simulink model "full_car_model"  (Simulink 7.0)
settings: Solver=ode45  StartTime=0.0  StopTime=120  RelTol=1e-3
values from neighbouring files (symbols this model uses):
  M = 0.02897    [CalculateTireWeight.m]    (also in SimFunc.m = [M11 M12; matrix_main.m)
undefined symbols (not defined in the file or in its folder): a, b, c, c01, c02, c03, c04, c1, c2, c3, c4, d, Ix, Iy, k01, k02, k03, k04, k1, k2, k3, k4, m1, m2, m3, m4, sigbuilder_block
(part 2 of 2)

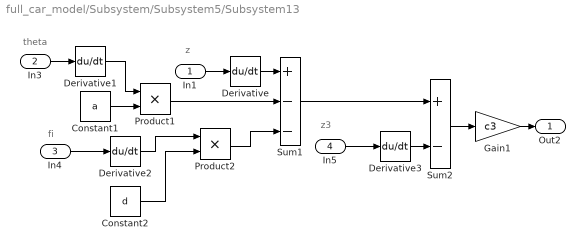
== system full_car_model/Subsystem/Subsystem5/Subsystem13 ==
  note: z3
  note: fi
  note: theta
  note: z
  In1 : Inport  OutDataType=sfix(16)  OutScaling=2^0
  In3 : Inport  Port=2  OutDataType=sfix(16)  OutScaling=2^0
  In4 : Inport  Port=3  OutDataType=sfix(16)  OutScaling=2^0
  In5 : Inport  Port=4  OutDataType=sfix(16)  OutScaling=2^0
  Constant1 : Constant  Value=a  OutDataType=sfix(16)  OutScaling=2^0
  Constant2 : Constant  Value=d  OutDataType=sfix(16)  OutScaling=2^0
  Derivative{,1..3} (4 alike) : Derivative
  Gain1 : Gain  Gain=c3  ParameterDataType=sfix(16)  ParameterScaling=2^0  OutDataType=sfix(16)  OutScaling=2^0
  Product1 : Product  OutDataType=sfix(16)  OutScaling=2^0  RndMeth=Zero
  Product2 : Product  OutDataType=sfix(16)  OutScaling=2^0  RndMeth=Zero
  Sum1 : Sum  Inputs=+--  OutDataType=sfix(16)  OutScaling=2^0
  Sum2 : Sum  Inputs=+-  OutDataType=sfix(16)  OutScaling=2^0
  Out2 : Outport  OutDataType=sfix(16)  OutScaling=2^0
  wires:
  Derivative2/1 -> Product2/1
  Derivative1/1 -> Product1/1
  Derivative/1 -> Sum1/1
  Gain1/1 -> Out2/1
  Product2/1 -> Sum1/3
  In5/1 -> Derivative3/1
  Constant2/1 -> Product2/2
  Product1/1 -> Sum1/2
  Constant1/1 -> Product1/2
  In4/1 -> Derivative2/1
  In3/1 -> Derivative1/1
  In1/1 -> Derivative/1
  Sum1/1 -> Sum2/1
  Derivative3/1 -> Sum2/2
  Sum2/1 -> Gain1/1

== system full_car_model/Subsystem/Subsystem6/Subsystem14 ==
  note: z4
  note: fi
  note: theta
  note: z
  In1 : Inport  OutDataType=sfix(16)  OutScaling=2^0
  In3 : Inport  Port=2  OutDataType=sfix(16)  OutScaling=2^0
  In4 : Inport  Port=3  OutDataType=sfix(16)  OutScaling=2^0
  In5 : Inport  Port=4  OutDataType=sfix(16)  OutScaling=2^0
  Constant1 : Constant  Value=b  OutDataType=sfix(16)  OutScaling=2^0
  Constant2 : Constant  Value=d  OutDataType=sfix(16)  OutScaling=2^0
  Gain1 : Gain  Gain=k4  ParameterDataType=sfix(16)  ParameterScaling=2^0  OutDataType=sfix(16)  OutScaling=2^0
  Product1 : Product  OutDataType=sfix(16)  OutScaling=2^0  RndMeth=Zero
  Product2 : Product  OutDataType=sfix(16)  OutScaling=2^0  RndMeth=Zero
  Sum1 : Sum  Inputs=++-  OutDataType=sfix(16)  OutScaling=2^0
  Sum2 : Sum  Inputs=+-  OutDataType=sfix(16)  OutScaling=2^0
  Out2 : Outport  OutDataType=sfix(16)  OutScaling=2^0
  wires:
  Gain1/1 -> Out2/1
  Product2/1 -> Sum1/3
  Constant2/1 -> Product2/2
  Product1/1 -> Sum1/2
  Constant1/1 -> Product1/2
  In4/1 -> Product2/1
  In3/1 -> Product1/1
  In1/1 -> Sum1/1
  Sum1/1 -> Sum2/1
  In5/1 -> Sum2/2
  Sum2/1 -> Gain1/1

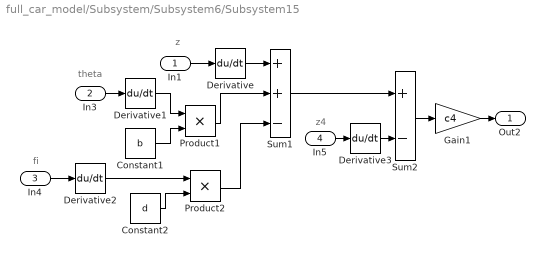
== system full_car_model/Subsystem/Subsystem6/Subsystem15 ==
  note: z
  note: theta
  note: fi
  note: z4
  In1 : Inport  OutDataType=sfix(16)  OutScaling=2^0
  In3 : Inport  Port=2  OutDataType=sfix(16)  OutScaling=2^0
  In4 : Inport  Port=3  OutDataType=sfix(16)  OutScaling=2^0
  In5 : Inport  Port=4  OutDataType=sfix(16)  OutScaling=2^0
  Constant1 : Constant  Value=b  OutDataType=sfix(16)  OutScaling=2^0
  Constant2 : Constant  Value=d  OutDataType=sfix(16)  OutScaling=2^0
  Derivative{,1..3} (4 alike) : Derivative
  Gain1 : Gain  Gain=c4  ParameterDataType=sfix(16)  ParameterScaling=2^0  OutDataType=sfix(16)  OutScaling=2^0
  Product1 : Product  OutDataType=sfix(16)  OutScaling=2^0  RndMeth=Zero
  Product2 : Product  OutDataType=sfix(16)  OutScaling=2^0  RndMeth=Zero
  Sum1 : Sum  Inputs=++-  OutDataType=sfix(16)  OutScaling=2^0
  Sum2 : Sum  Inputs=+-  OutDataType=sfix(16)  OutScaling=2^0
  Out2 : Outport  OutDataType=sfix(16)  OutScaling=2^0
  wires:
  Derivative2/1 -> Product2/1
  Derivative1/1 -> Product1/1
  Derivative/1 -> Sum1/1
  In1/1 -> Derivative/1
  In3/1 -> Derivative1/1
  In4/1 -> Derivative2/1
  Constant1/1 -> Product1/2
  Product1/1 -> Sum1/2
  Constant2/1 -> Product2/2
  In5/1 -> Derivative3/1
  Product2/1 -> Sum1/3
  Gain1/1 -> Out2/1
  Sum1/1 -> Sum2/1
  Derivative3/1 -> Sum2/2
  Sum2/1 -> Gain1/1

== system full_car_model/Subsystem1/Subsystem10/Subsystem20 ==
  note: z4
  note: fi
  note: theta
  note: z
  In1 : Inport  OutDataType=sfix(16)  OutScaling=2^0
  In3 : Inport  Port=2  OutDataType=sfix(16)  OutScaling=2^0
  In4 : Inport  Port=3  OutDataType=sfix(16)  OutScaling=2^0
  In5 : Inport  Port=4  OutDataType=sfix(16)  OutScaling=2^0
  Constant1 : Constant  Value=b  OutDataType=sfix(16)  OutScaling=2^0
  Constant2 : Constant  Value=d  OutDataType=sfix(16)  OutScaling=2^0
  Gain1 : Gain  Gain=k4  ParameterDataType=sfix(16)  ParameterScaling=2^0  OutDataType=sfix(16)  OutScaling=2^0
  Product1 : Product  OutDataType=sfix(16)  OutScaling=2^0  RndMeth=Zero
  Product2 : Product  OutDataType=sfix(16)  OutScaling=2^0  RndMeth=Zero
  Sum1 : Sum  Inputs=++-  OutDataType=sfix(16)  OutScaling=2^0
  Sum2 : Sum  Inputs=+-  OutDataType=sfix(16)  OutScaling=2^0
  Out2 : Outport  OutDataType=sfix(16)  OutScaling=2^0
  wires:
  Gain1/1 -> Out2/1
  Product2/1 -> Sum1/3
  Constant2/1 -> Product2/2
  Product1/1 -> Sum1/2
  Constant1/1 -> Product1/2
  In4/1 -> Product2/1
  In3/1 -> Product1/1
  In1/1 -> Sum1/1
  Sum1/1 -> Sum2/1
  In5/1 -> Sum2/2
  Sum2/1 -> Gain1/1

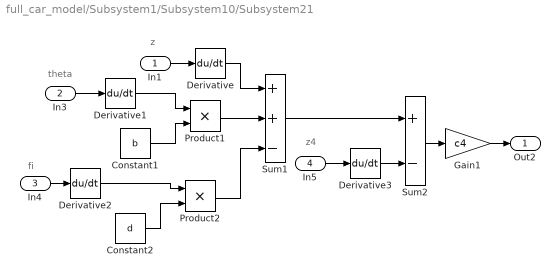
== system full_car_model/Subsystem1/Subsystem10/Subsystem21 ==
  note: z
  note: theta
  note: fi
  note: z4
  In1 : Inport  OutDataType=sfix(16)  OutScaling=2^0
  In3 : Inport  Port=2  OutDataType=sfix(16)  OutScaling=2^0
  In4 : Inport  Port=3  OutDataType=sfix(16)  OutScaling=2^0
  In5 : Inport  Port=4  OutDataType=sfix(16)  OutScaling=2^0
  Constant1 : Constant  Value=b  OutDataType=sfix(16)  OutScaling=2^0
  Constant2 : Constant  Value=d  OutDataType=sfix(16)  OutScaling=2^0
  Derivative{,1..3} (4 alike) : Derivative
  Gain1 : Gain  Gain=c4  ParameterDataType=sfix(16)  ParameterScaling=2^0  OutDataType=sfix(16)  OutScaling=2^0
  Product1 : Product  OutDataType=sfix(16)  OutScaling=2^0  RndMeth=Zero
  Product2 : Product  OutDataType=sfix(16)  OutScaling=2^0  RndMeth=Zero
  Sum1 : Sum  Inputs=++-  OutDataType=sfix(16)  OutScaling=2^0
  Sum2 : Sum  Inputs=+-  OutDataType=sfix(16)  OutScaling=2^0
  Out2 : Outport  OutDataType=sfix(16)  OutScaling=2^0
  wires:
  Derivative2/1 -> Product2/1
  Derivative1/1 -> Product1/1
  Derivative/1 -> Sum1/1
  In1/1 -> Derivative/1
  In3/1 -> Derivative1/1
  In4/1 -> Derivative2/1
  Constant1/1 -> Product1/2
  Product1/1 -> Sum1/2
  Constant2/1 -> Product2/2
  In5/1 -> Derivative3/1
  Product2/1 -> Sum1/3
  Gain1/1 -> Out2/1
  Sum1/1 -> Sum2/1
  Derivative3/1 -> Sum2/2
  Sum2/1 -> Gain1/1

== system full_car_model/Subsystem1/Subsystem7/Subsystem22 ==
  note: z1
  note: fi
  note: theta
  note: z
  In1 : Inport  OutDataType=sfix(16)  OutScaling=2^0
  In3 : Inport  Port=2  OutDataType=sfix(16)  OutScaling=2^0
  In4 : Inport  Port=3  OutDataType=sfix(16)  OutScaling=2^0
  In5 : Inport  Port=4  OutDataType=sfix(16)  OutScaling=2^0
  Constant1 : Constant  Value=a  OutDataType=sfix(16)  OutScaling=2^0
  Constant2 : Constant  Value=c  OutDataType=sfix(16)  OutScaling=2^0
  Gain1 : Gain  Gain=k1  ParameterDataType=sfix(16)  ParameterScaling=2^0  OutDataType=sfix(16)  OutScaling=2^0
  Product1 : Product  OutDataType=sfix(16)  OutScaling=2^0  RndMeth=Zero
  Product2 : Product  OutDataType=sfix(16)  OutScaling=2^0  RndMeth=Zero
  Sum1 : Sum  Inputs=+-+  OutDataType=sfix(16)  OutScaling=2^0
  Sum2 : Sum  Inputs=+-  OutDataType=sfix(16)  OutScaling=2^0
  Out2 : Outport  OutDataType=sfix(16)  OutScaling=2^0
  wires:
  Gain1/1 -> Out2/1
  Product2/1 -> Sum1/3
  Constant2/1 -> Product2/2
  Product1/1 -> Sum1/2
  Constant1/1 -> Product1/2
  In4/1 -> Product2/1
  In3/1 -> Product1/1
  In1/1 -> Sum1/1
  Sum1/1 -> Sum2/1
  In5/1 -> Sum2/2
  Sum2/1 -> Gain1/1

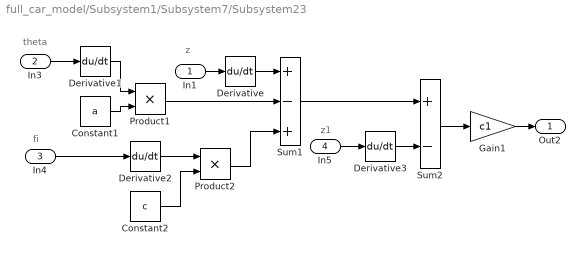
== system full_car_model/Subsystem1/Subsystem7/Subsystem23 ==
  note: z
  note: theta
  note: fi
  note: z1
  In1 : Inport  OutDataType=sfix(16)  OutScaling=2^0
  In3 : Inport  Port=2  OutDataType=sfix(16)  OutScaling=2^0
  In4 : Inport  Port=3  OutDataType=sfix(16)  OutScaling=2^0
  In5 : Inport  Port=4  OutDataType=sfix(16)  OutScaling=2^0
  Constant1 : Constant  Value=a  OutDataType=sfix(16)  OutScaling=2^0
  Constant2 : Constant  Value=c  OutDataType=sfix(16)  OutScaling=2^0
  Derivative{,1..3} (4 alike) : Derivative
  Gain1 : Gain  Gain=c1  ParameterDataType=sfix(16)  ParameterScaling=2^0  OutDataType=sfix(16)  OutScaling=2^0
  Product1 : Product  OutDataType=sfix(16)  OutScaling=2^0  RndMeth=Zero
  Product2 : Product  OutDataType=sfix(16)  OutScaling=2^0  RndMeth=Zero
  Sum1 : Sum  Inputs=+-+  OutDataType=sfix(16)  OutScaling=2^0
  Sum2 : Sum  Inputs=+-  OutDataType=sfix(16)  OutScaling=2^0
  Out2 : Outport  OutDataType=sfix(16)  OutScaling=2^0
  wires:
  Derivative2/1 -> Product2/1
  Derivative1/1 -> Product1/1
  Derivative/1 -> Sum1/1
  In1/1 -> Derivative/1
  In3/1 -> Derivative1/1
  In4/1 -> Derivative2/1
  Constant1/1 -> Product1/2
  Product1/1 -> Sum1/2
  Constant2/1 -> Product2/2
  In5/1 -> Derivative3/1
  Product2/1 -> Sum1/3
  Gain1/1 -> Out2/1
  Sum1/1 -> Sum2/1
  Derivative3/1 -> Sum2/2
  Sum2/1 -> Gain1/1

== system full_car_model/Subsystem1/Subsystem8/Subsystem16 ==
  note: z2
  note: fi
  note: theta
  note: z
  In1 : Inport  OutDataType=sfix(16)  OutScaling=2^0
  In3 : Inport  Port=2  OutDataType=sfix(16)  OutScaling=2^0
  In4 : Inport  Port=3  OutDataType=sfix(16)  OutScaling=2^0
  In5 : Inport  Port=4  OutDataType=sfix(16)  OutScaling=2^0
  Constant1 : Constant  Value=b  OutDataType=sfix(16)  OutScaling=2^0
  Constant2 : Constant  Value=c  OutDataType=sfix(16)  OutScaling=2^0
  Gain1 : Gain  Gain=k2  ParameterDataType=sfix(16)  ParameterScaling=2^0  OutDataType=sfix(16)  OutScaling=2^0
  Product1 : Product  OutDataType=sfix(16)  OutScaling=2^0  RndMeth=Zero
  Product2 : Product  OutDataType=sfix(16)  OutScaling=2^0  RndMeth=Zero
  Sum1 : Sum  Inputs=+++  OutDataType=sfix(16)  OutScaling=2^0
  Sum2 : Sum  Inputs=+-  OutDataType=sfix(16)  OutScaling=2^0
  Out2 : Outport  OutDataType=sfix(16)  OutScaling=2^0
  wires:
  Gain1/1 -> Out2/1
  Product2/1 -> Sum1/3
  Constant2/1 -> Product2/2
  Product1/1 -> Sum1/2
  Constant1/1 -> Product1/2
  In4/1 -> Product2/1
  In3/1 -> Product1/1
  In1/1 -> Sum1/1
  Sum1/1 -> Sum2/1
  In5/1 -> Sum2/2
  Sum2/1 -> Gain1/1

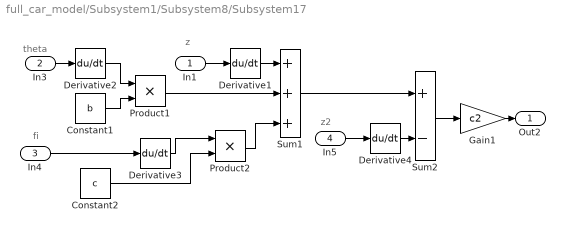
== system full_car_model/Subsystem1/Subsystem8/Subsystem17 ==
  note: z
  note: theta
  note: fi
  note: z2
  In1 : Inport  OutDataType=sfix(16)  OutScaling=2^0
  In3 : Inport  Port=2  OutDataType=sfix(16)  OutScaling=2^0
  In4 : Inport  Port=3  OutDataType=sfix(16)  OutScaling=2^0
  In5 : Inport  Port=4  OutDataType=sfix(16)  OutScaling=2^0
  Constant1 : Constant  Value=b  OutDataType=sfix(16)  OutScaling=2^0
  Constant2 : Constant  Value=c  OutDataType=sfix(16)  OutScaling=2^0
  Derivative{1..4} (4 alike) : Derivative
  Gain1 : Gain  Gain=c2  ParameterDataType=sfix(16)  ParameterScaling=2^0  OutDataType=sfix(16)  OutScaling=2^0
  Product1 : Product  OutDataType=sfix(16)  OutScaling=2^0  RndMeth=Zero
  Product2 : Product  OutDataType=sfix(16)  OutScaling=2^0  RndMeth=Zero
  Sum1 : Sum  Inputs=+++  OutDataType=sfix(16)  OutScaling=2^0
  Sum2 : Sum  Inputs=+-  OutDataType=sfix(16)  OutScaling=2^0
  Out2 : Outport  OutDataType=sfix(16)  OutScaling=2^0
  wires:
  Derivative3/1 -> Product2/1
  Derivative2/1 -> Product1/1
  Derivative1/1 -> Sum1/1
  In1/1 -> Derivative1/1
  In3/1 -> Derivative2/1
  In4/1 -> Derivative3/1
  Constant1/1 -> Product1/2
  Product1/1 -> Sum1/2
  Constant2/1 -> Product2/2
  In5/1 -> Derivative4/1
  Product2/1 -> Sum1/3
  Gain1/1 -> Out2/1
  Sum1/1 -> Sum2/1
  Derivative4/1 -> Sum2/2
  Sum2/1 -> Gain1/1

== system full_car_model/Subsystem1/Subsystem9/Subsystem18 ==
  note: z
  note: theta
  note: fi
  note: z3
  In1 : Inport  OutDataType=sfix(16)  OutScaling=2^0
  In3 : Inport  Port=2  OutDataType=sfix(16)  OutScaling=2^0
  In4 : Inport  Port=3  OutDataType=sfix(16)  OutScaling=2^0
  In5 : Inport  Port=4  OutDataType=sfix(16)  OutScaling=2^0
  Constant1 : Constant  Value=a  OutDataType=sfix(16)  OutScaling=2^0
  Constant2 : Constant  Value=d  OutDataType=sfix(16)  OutScaling=2^0
  Gain1 : Gain  Gain=k3  ParameterDataType=sfix(16)  ParameterScaling=2^0  OutDataType=sfix(16)  OutScaling=2^0
  Product1 : Product  OutDataType=sfix(16)  OutScaling=2^0  RndMeth=Zero
  Product2 : Product  OutDataType=sfix(16)  OutScaling=2^0  RndMeth=Zero
  Sum1 : Sum  Inputs=+--  OutDataType=sfix(16)  OutScaling=2^0
  Sum2 : Sum  Inputs=+-  OutDataType=sfix(16)  OutScaling=2^0
  Out2 : Outport  OutDataType=sfix(16)  OutScaling=2^0
  wires:
  In1/1 -> Sum1/1
  In3/1 -> Product1/1
  In4/1 -> Product2/1
  Constant1/1 -> Product1/2
  Product1/1 -> Sum1/2
  Constant2/1 -> Product2/2
  Product2/1 -> Sum1/3
  Gain1/1 -> Out2/1
  Sum1/1 -> Sum2/1
  In5/1 -> Sum2/2
  Sum2/1 -> Gain1/1

== system full_car_model/Subsystem1/Subsystem9/Subsystem19 ==
  note: z3
  note: fi
  note: theta
  note: z
  In1 : Inport  OutDataType=sfix(16)  OutScaling=2^0
  In3 : Inport  Port=2  OutDataType=sfix(16)  OutScaling=2^0
  In4 : Inport  Port=3  OutDataType=sfix(16)  OutScaling=2^0
  In5 : Inport  Port=4  OutDataType=sfix(16)  OutScaling=2^0
  Constant1 : Constant  Value=a  OutDataType=sfix(16)  OutScaling=2^0
  Constant2 : Constant  Value=d  OutDataType=sfix(16)  OutScaling=2^0
  Derivative{,1..3} (4 alike) : Derivative
  Gain1 : Gain  Gain=c3  ParameterDataType=sfix(16)  ParameterScaling=2^0  OutDataType=sfix(16)  OutScaling=2^0
  Product1 : Product  OutDataType=sfix(16)  OutScaling=2^0  RndMeth=Zero
  Product2 : Product  OutDataType=sfix(16)  OutScaling=2^0  RndMeth=Zero
  Sum1 : Sum  Inputs=+--  OutDataType=sfix(16)  OutScaling=2^0
  Sum2 : Sum  Inputs=+-  OutDataType=sfix(16)  OutScaling=2^0
  Out2 : Outport  OutDataType=sfix(16)  OutScaling=2^0
  wires:
  Derivative2/1 -> Product2/1
  Derivative1/1 -> Product1/1
  Derivative/1 -> Sum1/1
  Gain1/1 -> Out2/1
  Product2/1 -> Sum1/3
  In5/1 -> Derivative3/1
  Constant2/1 -> Product2/2
  Product1/1 -> Sum1/2
  Constant1/1 -> Product1/2
  In4/1 -> Derivative2/1
  In3/1 -> Derivative1/1
  In1/1 -> Derivative/1
  Sum1/1 -> Sum2/1
  Derivative3/1 -> Sum2/2
  Sum2/1 -> Gain1/1

== system full_car_model/Subsystem11/Subsystem/Subsystem2 ==
  note: z
  note: theta
  note: fi
  note: z2
  In1 : Inport  OutDataType=sfix(16)  OutScaling=2^0
  In3 : Inport  Port=2  OutDataType=sfix(16)  OutScaling=2^0
  In4 : Inport  Port=3  OutDataType=sfix(16)  OutScaling=2^0
  In5 : Inport  Port=4  OutDataType=sfix(16)  OutScaling=2^0
  Constant1 : Constant  Value=b  OutDataType=sfix(16)  OutScaling=2^0
  Constant2 : Constant  Value=c  OutDataType=sfix(16)  OutScaling=2^0
  Gain1 : Gain  Gain=k2  ParameterDataType=sfix(16)  ParameterScaling=2^0  OutDataType=sfix(16)  OutScaling=2^0
  Product1 : Product  OutDataType=sfix(16)  OutScaling=2^0  RndMeth=Zero
  Product2 : Product  OutDataType=sfix(16)  OutScaling=2^0  RndMeth=Zero
  Sum1 : Sum  Inputs=+++  OutDataType=sfix(16)  OutScaling=2^0
  Sum2 : Sum  Inputs=+-  OutDataType=sfix(16)  OutScaling=2^0
  Out2 : Outport  OutDataType=sfix(16)  OutScaling=2^0
  wires:
  In1/1 -> Sum1/1
  In3/1 -> Product1/1
  In4/1 -> Product2/1
  Constant1/1 -> Product1/2
  Product1/1 -> Sum1/2
  Constant2/1 -> Product2/2
  Product2/1 -> Sum1/3
  Gain1/1 -> Out2/1
  Sum1/1 -> Sum2/1
  In5/1 -> Sum2/2
  Sum2/1 -> Gain1/1

== system full_car_model/Subsystem11/Subsystem/Subsystem3 ==
  note: z2
  note: fi
  note: theta
  note: z
  In1 : Inport  OutDataType=sfix(16)  OutScaling=2^0
  In3 : Inport  Port=2  OutDataType=sfix(16)  OutScaling=2^0
  In4 : Inport  Port=3  OutDataType=sfix(16)  OutScaling=2^0
  In5 : Inport  Port=4  OutDataType=sfix(16)  OutScaling=2^0
  Constant1 : Constant  Value=b  OutDataType=sfix(16)  OutScaling=2^0
  Constant2 : Constant  Value=c  OutDataType=sfix(16)  OutScaling=2^0
  Derivative{1..4} (4 alike) : Derivative
  Gain1 : Gain  Gain=c2  ParameterDataType=sfix(16)  ParameterScaling=2^0  OutDataType=sfix(16)  OutScaling=2^0
  Product1 : Product  OutDataType=sfix(16)  OutScaling=2^0  RndMeth=Zero
  Product2 : Product  OutDataType=sfix(16)  OutScaling=2^0  RndMeth=Zero
  Sum1 : Sum  Inputs=+++  OutDataType=sfix(16)  OutScaling=2^0
  Sum2 : Sum  Inputs=+-  OutDataType=sfix(16)  OutScaling=2^0
  Out2 : Outport  OutDataType=sfix(16)  OutScaling=2^0
  wires:
  Gain1/1 -> Out2/1
  Product2/1 -> Sum1/3
  In5/1 -> Derivative4/1
  Constant2/1 -> Product2/2
  Product1/1 -> Sum1/2
  Constant1/1 -> Product1/2
  In4/1 -> Derivative3/1
  In3/1 -> Derivative2/1
  In1/1 -> Derivative1/1
  Derivative1/1 -> Sum1/1
  Derivative2/1 -> Product1/1
  Derivative3/1 -> Product2/1
  Sum1/1 -> Sum2/1
  Sum2/1 -> Gain1/1
  Derivative4/1 -> Sum2/2

== system full_car_model/Subsystem11/Subsystem1/Subsystem4 ==
  note: z3
  note: fi
  note: theta
  note: z
  In1 : Inport  OutDataType=sfix(16)  OutScaling=2^0
  In3 : Inport  Port=2  OutDataType=sfix(16)  OutScaling=2^0
  In4 : Inport  Port=3  OutDataType=sfix(16)  OutScaling=2^0
  In5 : Inport  Port=4  OutDataType=sfix(16)  OutScaling=2^0
  Constant1 : Constant  Value=a  OutDataType=sfix(16)  OutScaling=2^0
  Constant2 : Constant  Value=d  OutDataType=sfix(16)  OutScaling=2^0
  Gain1 : Gain  Gain=k3  ParameterDataType=sfix(16)  ParameterScaling=2^0  OutDataType=sfix(16)  OutScaling=2^0
  Product1 : Product  OutDataType=sfix(16)  OutScaling=2^0  RndMeth=Zero
  Product2 : Product  OutDataType=sfix(16)  OutScaling=2^0  RndMeth=Zero
  Sum1 : Sum  Inputs=+--  OutDataType=sfix(16)  OutScaling=2^0
  Sum2 : Sum  Inputs=+-  OutDataType=sfix(16)  OutScaling=2^0
  Out2 : Outport  OutDataType=sfix(16)  OutScaling=2^0
  wires:
  Gain1/1 -> Out2/1
  Product2/1 -> Sum1/3
  Constant2/1 -> Product2/2
  Product1/1 -> Sum1/2
  Constant1/1 -> Product1/2
  In4/1 -> Product2/1
  In3/1 -> Product1/1
  In1/1 -> Sum1/1
  In5/1 -> Sum2/2
  Sum1/1 -> Sum2/1
  Sum2/1 -> Gain1/1

== system full_car_model/Subsystem11/Subsystem1/Subsystem5 ==
  note: z
  note: theta
  note: fi
  note: z3
  In1 : Inport  OutDataType=sfix(16)  OutScaling=2^0
  In3 : Inport  Port=2  OutDataType=sfix(16)  OutScaling=2^0
  In4 : Inport  Port=3  OutDataType=sfix(16)  OutScaling=2^0
  In5 : Inport  Port=4  OutDataType=sfix(16)  OutScaling=2^0
  Constant1 : Constant  Value=a  OutDataType=sfix(16)  OutScaling=2^0
  Constant2 : Constant  Value=d  OutDataType=sfix(16)  OutScaling=2^0
  Derivative{,1..3} (4 alike) : Derivative
  Gain1 : Gain  Gain=c3  ParameterDataType=sfix(16)  ParameterScaling=2^0  OutDataType=sfix(16)  OutScaling=2^0
  Product1 : Product  OutDataType=sfix(16)  OutScaling=2^0  RndMeth=Zero
  Product2 : Product  OutDataType=sfix(16)  OutScaling=2^0  RndMeth=Zero
  Sum1 : Sum  Inputs=+--  OutDataType=sfix(16)  OutScaling=2^0
  Sum2 : Sum  Inputs=+-  OutDataType=sfix(16)  OutScaling=2^0
  Out2 : Outport  OutDataType=sfix(16)  OutScaling=2^0
  wires:
  In1/1 -> Derivative/1
  In3/1 -> Derivative1/1
  In4/1 -> Derivative2/1
  Constant1/1 -> Product1/2
  Product1/1 -> Sum1/2
  Constant2/1 -> Product2/2
  In5/1 -> Derivative3/1
  Product2/1 -> Sum1/3
  Gain1/1 -> Out2/1
  Derivative/1 -> Sum1/1
  Derivative1/1 -> Product1/1
  Derivative2/1 -> Product2/1
  Derivative3/1 -> Sum2/2
  Sum2/1 -> Gain1/1
  Sum1/1 -> Sum2/1

== system full_car_model/Subsystem11/Subsystem2/Subsystem6 ==
  note: z
  note: theta
  note: fi
  note: z4
  In1 : Inport  OutDataType=sfix(16)  OutScaling=2^0
  In3 : Inport  Port=2  OutDataType=sfix(16)  OutScaling=2^0
  In4 : Inport  Port=3  OutDataType=sfix(16)  OutScaling=2^0
  In5 : Inport  Port=4  OutDataType=sfix(16)  OutScaling=2^0
  Constant1 : Constant  Value=b  OutDataType=sfix(16)  OutScaling=2^0
  Constant2 : Constant  Value=d  OutDataType=sfix(16)  OutScaling=2^0
  Gain1 : Gain  Gain=k4  ParameterDataType=sfix(16)  ParameterScaling=2^0  OutDataType=sfix(16)  OutScaling=2^0
  Product1 : Product  OutDataType=sfix(16)  OutScaling=2^0  RndMeth=Zero
  Product2 : Product  OutDataType=sfix(16)  OutScaling=2^0  RndMeth=Zero
  Sum1 : Sum  Inputs=++-  OutDataType=sfix(16)  OutScaling=2^0
  Sum2 : Sum  Inputs=+-  OutDataType=sfix(16)  OutScaling=2^0
  Out2 : Outport  OutDataType=sfix(16)  OutScaling=2^0
  wires:
  In1/1 -> Sum1/1
  In3/1 -> Product1/1
  In4/1 -> Product2/1
  Constant1/1 -> Product1/2
  Product1/1 -> Sum1/2
  Constant2/1 -> Product2/2
  Product2/1 -> Sum1/3
  Gain1/1 -> Out2/1
  In5/1 -> Sum2/2
  Sum1/1 -> Sum2/1
  Sum2/1 -> Gain1/1

== system full_car_model/Subsystem11/Subsystem2/Subsystem7 ==
  note: z4
  note: fi
  note: theta
  note: z
  In1 : Inport  OutDataType=sfix(16)  OutScaling=2^0
  In3 : Inport  Port=2  OutDataType=sfix(16)  OutScaling=2^0
  In4 : Inport  Port=3  OutDataType=sfix(16)  OutScaling=2^0
  In5 : Inport  Port=4  OutDataType=sfix(16)  OutScaling=2^0
  Constant1 : Constant  Value=b  OutDataType=sfix(16)  OutScaling=2^0
  Constant2 : Constant  Value=d  OutDataType=sfix(16)  OutScaling=2^0
  Derivative{,1..3} (4 alike) : Derivative
  Gain1 : Gain  Gain=c4  ParameterDataType=sfix(16)  ParameterScaling=2^0  OutDataType=sfix(16)  OutScaling=2^0
  Product1 : Product  OutDataType=sfix(16)  OutScaling=2^0  RndMeth=Zero
  Product2 : Product  OutDataType=sfix(16)  OutScaling=2^0  RndMeth=Zero
  Sum1 : Sum  Inputs=++-  OutDataType=sfix(16)  OutScaling=2^0
  Sum2 : Sum  Inputs=+-  OutDataType=sfix(16)  OutScaling=2^0
  Out2 : Outport  OutDataType=sfix(16)  OutScaling=2^0
  wires:
  Gain1/1 -> Out2/1
  Product2/1 -> Sum1/3
  In5/1 -> Derivative3/1
  Constant2/1 -> Product2/2
  Product1/1 -> Sum1/2
  Constant1/1 -> Product1/2
  In4/1 -> Derivative2/1
  In3/1 -> Derivative1/1
  In1/1 -> Derivative/1
  Derivative/1 -> Sum1/1
  Derivative1/1 -> Product1/1
  Derivative2/1 -> Product2/1
  Derivative3/1 -> Sum2/2
  Sum1/1 -> Sum2/1
  Sum2/1 -> Gain1/1

== system full_car_model/Subsystem11/Subsystem40/Subsystem ==
  note: z
  note: theta
  note: fi
  note: z1
  In1 : Inport  OutDataType=sfix(16)  OutScaling=2^0
  In3 : Inport  Port=2  OutDataType=sfix(16)  OutScaling=2^0
  In4 : Inport  Port=3  OutDataType=sfix(16)  OutScaling=2^0
  In5 : Inport  Port=4  OutDataType=sfix(16)  OutScaling=2^0
  Constant1 : Constant  Value=a  OutDataType=sfix(16)  OutScaling=2^0
  Constant2 : Constant  Value=c  OutDataType=sfix(16)  OutScaling=2^0
  Gain1 : Gain  Gain=k1  ParameterDataType=sfix(16)  ParameterScaling=2^0  OutDataType=sfix(16)  OutScaling=2^0
  Product1 : Product  OutDataType=sfix(16)  OutScaling=2^0  RndMeth=Zero
  Product2 : Product  OutDataType=sfix(16)  OutScaling=2^0  RndMeth=Zero
  Sum1 : Sum  Inputs=+-+  OutDataType=sfix(16)  OutScaling=2^0
  Sum2 : Sum  Inputs=+-  OutDataType=sfix(16)  OutScaling=2^0
  Out2 : Outport  OutDataType=sfix(16)  OutScaling=2^0
  wires:
  In1/1 -> Sum1/1
  In3/1 -> Product1/1
  In4/1 -> Product2/1
  Constant1/1 -> Product1/2
  Product1/1 -> Sum1/2
  Constant2/1 -> Product2/2
  Product2/1 -> Sum1/3
  Gain1/1 -> Out2/1
  Sum1/1 -> Sum2/1
  In5/1 -> Sum2/2
  Sum2/1 -> Gain1/1

== system full_car_model/Subsystem11/Subsystem40/Subsystem1 ==
  note: z1
  note: fi
  note: theta
  note: z
  In1 : Inport  OutDataType=sfix(16)  OutScaling=2^0
  In3 : Inport  Port=2  OutDataType=sfix(16)  OutScaling=2^0
  In4 : Inport  Port=3  OutDataType=sfix(16)  OutScaling=2^0
  In5 : Inport  Port=4  OutDataType=sfix(16)  OutScaling=2^0
  Constant1 : Constant  Value=a  OutDataType=sfix(16)  OutScaling=2^0
  Constant2 : Constant  Value=c  OutDataType=sfix(16)  OutScaling=2^0
  Derivative{,1..3} (4 alike) : Derivative
  Gain1 : Gain  Gain=c1  ParameterDataType=sfix(16)  ParameterScaling=2^0  OutDataType=sfix(16)  OutScaling=2^0
  Product1 : Product  OutDataType=sfix(16)  OutScaling=2^0  RndMeth=Zero
  Product2 : Product  OutDataType=sfix(16)  OutScaling=2^0  RndMeth=Zero
  Sum1 : Sum  Inputs=+-+  OutDataType=sfix(16)  OutScaling=2^0
  Sum2 : Sum  Inputs=+-  OutDataType=sfix(16)  OutScaling=2^0
  Out2 : Outport  OutDataType=sfix(16)  OutScaling=2^0
  wires:
  Gain1/1 -> Out2/1
  Product2/1 -> Sum1/3
  In5/1 -> Derivative3/1
  Constant2/1 -> Product2/2
  Product1/1 -> Sum1/2
  Constant1/1 -> Product1/2
  In4/1 -> Derivative2/1
  In3/1 -> Derivative1/1
  In1/1 -> Derivative/1
  Derivative/1 -> Sum1/1
  Derivative1/1 -> Product1/1
  Derivative2/1 -> Product2/1
  Derivative3/1 -> Sum2/2
  Sum2/1 -> Gain1/1
  Sum1/1 -> Sum2/1
